simulink model "AltitudeControl"  (Simulink 7.2)
settings: Solver=ode45  StartTime=0.0  StopTime=10.0  RelTol=1e-3
undefined symbols (not defined in the file): DiscIntNeverNeededParam
settings Model: Creator=teme  LastModifiedBy=arnaud
settings OptimizationCC: ExpressionDepthLimit=128
settings DebuggingCC: FcnCallInpInsideContextMsg=Enable All  StrictBusMsg=ErrorLevel1
settings CodeAppCC: CustomSymbolStrType=$N$R$M_T

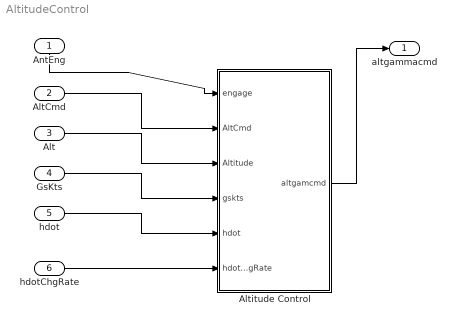
== system AltitudeControl ==
  AntEng : Inport  Orientation=down  DataType=boolean  OutDataTypeStr=boolean
  AltCmd : Inport  Port=2  DataType=double  OutDataTypeStr=double
  Alt : Inport  Port=3  DataType=double  OutDataTypeStr=double
  GsKts : Inport  Port=4  DataType=double  OutDataTypeStr=double
  hdot : Inport  Port=5  DataType=double  OutDataTypeStr=double
  hdotChgRate : Inport  Port=6  DataType=double  OutDataTypeStr=double
  Altitude Control : Subsystem  RequirementInfo={'other' '..\..\tcm_requirements.docx' '@Simulink_requirement_item_14' 'true' 'Altitude Control' '' } %GIDa_5c8df5fb_afa0_485e_88ca_9eaabd9d0f8f
  altgammacmd : Outport
  wires:
  Alt/1 -> Altitude Control/3(Altitude)
  AltCmd/1 -> Altitude Control/2(AltCmd)
  Altitude Control/1(altgamcmd) -> altgammacmd/1
  hdot/1 -> Altitude Control/5(hdot)
  GsKts/1 -> Altitude Control/4(gskts)
  AntEng/1 -> Altitude Control/1(engage)
  hdotChgRate/1 -> Altitude Control/6(hdotChgRate)

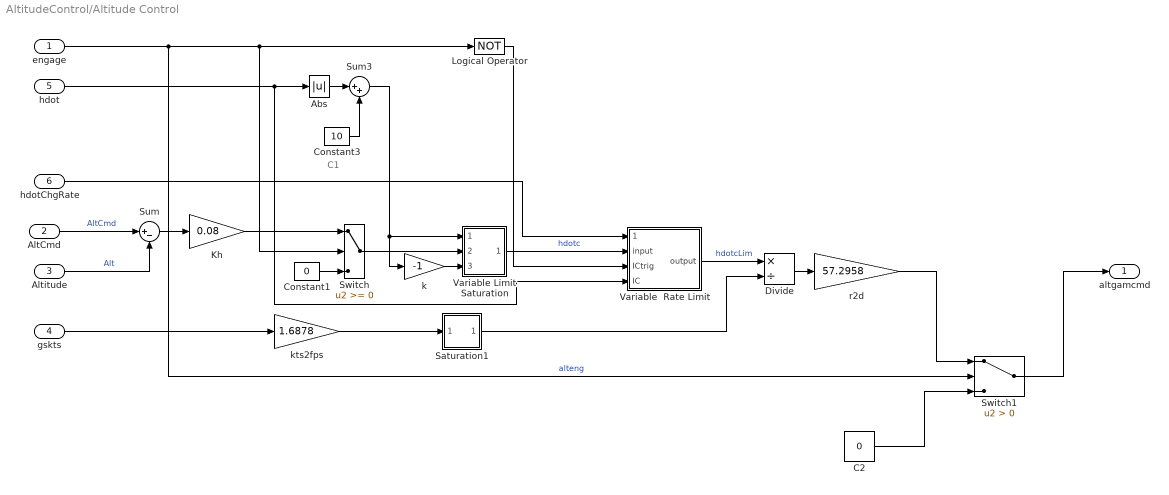
== system AltitudeControl/Altitude Control ==
  note: C1
  engage : Inport  RequirementInfo={} %GIDa_0e288978_810b_404d_8e3d_cfce00b6b13e
  AltCmd : Inport  RequirementInfo={} %GIDa_0cb28106_5eef_4f57_b895_6f6cc316bc91  Port=2
  Altitude : Inport  RequirementInfo={} %GIDa_9d659266_d3a1_41f7_8443_512a58352a3d  Port=3
  gskts : Inport  RequirementInfo={} %GIDa_63cbdc79_cc3a_41e8_a25c_03f8123eb444  Port=4
  hdot : Inport  RequirementInfo={} %GIDa_f80cf171_2707_4e4f_8e83_784456bc38b4  Port=5
  hdotChgRate : Inport  Port=6
  Abs : Abs  RequirementInfo={} %GIDa_20990742_0e4c_4a42_9d74_05382c3e5e10  SaturateOnIntegerOverflow=on
  C2 : Constant  Value=0
  Constant1 : Constant  RequirementInfo={} %GIDa_dca6c410_f388_4f73_ad77_90690c1c79ec  Value=0
  Constant3 : Constant  RequirementInfo={} %GIDa_4d484c55_e80b_4edf_b935_4d0b84fcef43  Value=10
  Divide : Product  RequirementInfo={} %GIDa_a21511b8_8e46_4269_9008_ba9a73618299  Inputs=*/
  Kh : Gain  RequirementInfo={} %GIDa_78bba325_b998_4ee3_b904_8fb0a7f7f7a7  Gain=0.08
  Logical Operator : Logic  RequirementInfo={} %GIDa_3db4e860_846f_470a_babf_a996fcc4fa8f  Operator=NOT
  Saturation1 : Subsystem  RequirementInfo={} %GIDa_f2f227d4_0c3d_4202_a816_beb06b8fee84  TreatAsAtomicUnit=on
  Sum : Sum  RequirementInfo={} %GIDa_c2c23c63_6291_4bac_a67f_cece50fd07b3  Inputs=|+-
  Sum3 : Sum  RequirementInfo={} %GIDa_abda5f80_1075_4cc6_bfe7_9e1cade77fe9  Inputs=|++  SaturateOnIntegerOverflow=on  InputSameDT=on  OutDataTypeStr=Inherit: Same as first input
  Switch : Switch  RequirementInfo={} %GIDa_a81bded5_11a5_4d9b_8d99_08187593493d
  Switch1 : Switch  Criteria=u2 > Threshold
  Variable  Rate Limit : Subsystem  RequirementInfo={} %GIDa_ca745fb3_1ac0_4f87_9ddc_ec0222d57c6c  TreatAsAtomicUnit=on
  Variable Limit Saturation : Subsystem  RequirementInfo={} %GIDa_ceaf2ff3_d3d5_4139_ac40_0e8f5fb26a06  TreatAsAtomicUnit=on
  k : Gain  RequirementInfo={} %GIDa_44367ca2_97f6_4cb9_9c49_9c779fdc721d  Gain=-1
  kts2fps : Gain  RequirementInfo={} %GIDa_8207b08e_fddf_4c38_87c9_e2cb216813f3  Gain=1.6878
  r2d : Gain  RequirementInfo={} %GIDa_573f61a6_cdca_472b_9b49_60142d70b114  Gain=57.2958
  altgamcmd : Outport  RequirementInfo={} %GIDa_cfdf8567_1bf1_487f_8025_1fae61c9e97a
  wires:
  Sum/1 -> Kh/1
  AltCmd/1 -> Sum/1  "AltCmd"
  Altitude/1 -> Sum/2  "Alt"
  hdot/1 -> Variable  Rate Limit/4(IC), Abs/1
  Abs/1 -> Sum3/1
  Constant3/1 -> Sum3/2
  k/1 -> Variable Limit Saturation/3(Lo_lim)
  Sum3/1 -> k/1, Variable Limit Saturation/1(up_lim)
  engage/1 -> Switch1/2, Switch/2, Logical Operator/1  "alteng"
  gskts/1 -> kts2fps/1
  Divide/1 -> r2d/1
  r2d/1 -> Switch1/1
  Logical Operator/1 -> Variable  Rate Limit/3(ICtrig)
  Variable Limit Saturation/1(Out1) -> Variable  Rate Limit/2(input)  "hdotc"
  hdotChgRate/1 -> Variable  Rate Limit/1(ratelim)
  Variable  Rate Limit/1(output) -> Divide/1  "hdotcLim"
  kts2fps/1 -> Saturation1/1(SigIn)
  Saturation1/1(Out1) -> Divide/2
  Switch/1 -> Variable Limit Saturation/2(SigIn)
  Kh/1 -> Switch/1
  Constant1/1 -> Switch/3
  Switch1/1 -> altgamcmd/1
  C2/1 -> Switch1/3

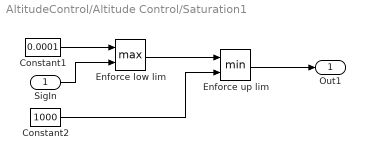
== system AltitudeControl/Altitude Control/Saturation1 ==
  SigIn : Inport  RequirementInfo={} %GIDa_3f5a5311_8185_423f_bf45_67fce5708cdf
  Constant1 : Constant  RequirementInfo={} %GIDa_5a314e61_37a6_49c9_8286_17afee39489d  Value=0.0001
  Constant2 : Constant  RequirementInfo={} %GIDa_19bb776a_128d_4f79_8f32_c6db1286f54e  Value=1000
  Enforce low lim : MinMax  RequirementInfo={} %GIDa_f1ed7bfa_f6af_4dde_ac1b_3ccc756e151e  Function=max  Inputs=2
  Enforce up lim : MinMax  RequirementInfo={} %GIDa_b7d41d07_03e7_4646_9c0d_3c39819752e0  Inputs=2
  Out1 : Outport  RequirementInfo={} %GIDa_a8215b4d_1c2e_47f3_a8fe_a5ea2625158e
  wires:
  Constant1/1 -> Enforce low lim/1
  SigIn/1 -> Enforce low lim/2
  Enforce low lim/1 -> Enforce up lim/1
  Constant2/1 -> Enforce up lim/2
  Enforce up lim/1 -> Out1/1

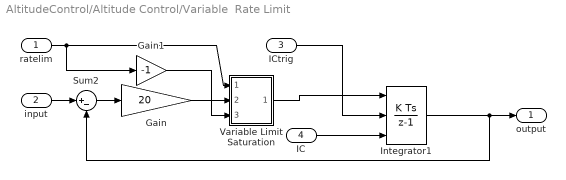
== system AltitudeControl/Altitude Control/Variable  Rate Limit ==
  ratelim : Inport  RequirementInfo={} %GIDa_8a409414_085c_4019_8b8a_edbb028e09c9
  input : Inport  RequirementInfo={} %GIDa_36ca4060_62d0_4794_bfac_efaeb948570f  Port=2  DataType=double  OutDataTypeStr=double
  ICtrig : Inport  RequirementInfo={} %GIDa_210448ec_8901_4d8b_9ae7_bf6603d5175a  Port=3
  IC : Inport  RequirementInfo={} %GIDa_ed78ca41_0e9a_442c_9ce9_efe3f633ea2f  Port=4
  Gain : Gain  RequirementInfo={} %GIDa_8ea2875b_9460_4c83_af15_3f6a067463fd  Gain=20  SaturateOnIntegerOverflow=on  OutDataTypeStr=Inherit: Same as input  ParamDataTypeStr=Inherit: Same as input
  Gain1 : Gain  RequirementInfo={} %GIDa_d92d949d_b0f7_438c_933d_85950dded665  Gain=-1  SaturateOnIntegerOverflow=on  OutDataTypeStr=Inherit: Same as input  ParamDataTypeStr=Inherit: Same as input
  Integrator1 : DiscreteIntegrator  ExternalReset=level  InitialConditionSource=external  SampleTime=0.1  ICPrevOutput=DiscIntNeverNeededParam  ICPrevScaledInput=DiscIntNeverNeededParam  mask(DiscretizedDiscreteIntegrator){}
      mask init:
      | %zoh
  Sum2 : Sum  RequirementInfo={} %GIDa_b334e623_37fe_4ac9_8a97_87088e45dc39  Inputs=|+-  SaturateOnIntegerOverflow=on
  Variable Limit Saturation : Subsystem  RequirementInfo={} %GIDa_455ee4b2_c105_48a1_b2ff_6f4ef26a2acf  TreatAsAtomicUnit=on
  output : Outport  RequirementInfo={} %GIDa_986bb623_f504_4c3d_99b4_2d7370fadfb9
  wires:
  Sum2/1 -> Gain/1
  Gain/1 -> Variable Limit Saturation/2(SigIn)
  ratelim/1 -> Gain1/1, Variable Limit Saturation/1(up_lim)
  Gain1/1 -> Variable Limit Saturation/3(Lo_lim)
  Integrator1/1 -> Sum2/2, output/1
  input/1 -> Sum2/1
  ICtrig/1 -> Integrator1/2
  IC/1 -> Integrator1/3
  Variable Limit Saturation/1(Out1) -> Integrator1/1

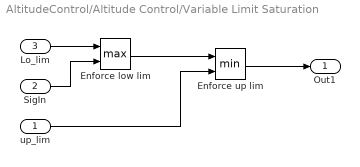
== system AltitudeControl/Altitude Control/Variable Limit Saturation ==
  up_lim : Inport  RequirementInfo={} %GIDa_2e88107a_170e_4209_87ba_bbf099e30048
  SigIn : Inport  RequirementInfo={} %GIDa_1009f7fd_18d1_47a6_bfe8_961b0527e63f  Port=2
  Lo_lim : Inport  RequirementInfo={} %GIDa_25d3a119_7934_4f14_885f_e425c054d3b7  Port=3
  Enforce low lim : MinMax  RequirementInfo={} %GIDa_569de777_726d_4b4c_9368_c3dc4036e8ed  Function=max  Inputs=2
  Enforce up lim : MinMax  RequirementInfo={} %GIDa_08ef4c7c_041a_47cf_8bce_d060e85fd321  Inputs=2
  Out1 : Outport  RequirementInfo={} %GIDa_e97969f5_319c_4569_953d_3be8dc8cd68b
  wires:
  Lo_lim/1 -> Enforce low lim/1
  SigIn/1 -> Enforce low lim/2
  Enforce low lim/1 -> Enforce up lim/1
  up_lim/1 -> Enforce up lim/2
  Enforce up lim/1 -> Out1/1

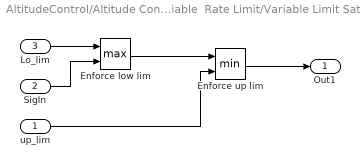
== system AltitudeControl/Altitude Control/Variable  Rate Limit/Variable Limit Saturation ==
  up_lim : Inport  RequirementInfo={} %GIDa_253765a1_7361_4d78_8d4d_1b11f15ce2fa
  SigIn : Inport  RequirementInfo={} %GIDa_df6737d0_f7fe_4781_af6c_3ea749d3e5de  Port=2
  Lo_lim : Inport  RequirementInfo={} %GIDa_c8822ea1_e967_4622_a20b_57b5cefb7799  Port=3
  Enforce low lim : MinMax  RequirementInfo={} %GIDa_fd2a26e9_6c43_40d9_92a2_3b773c237580  Function=max  Inputs=2
  Enforce up lim : MinMax  RequirementInfo={} %GIDa_ef782b40_f42e_44f8_8e6f_8bce9bd7a3f3  Inputs=2
  Out1 : Outport  RequirementInfo={} %GIDa_dbecd57e_14da_4974_8aa6_dc0e6b8a6b18
  wires:
  Enforce up lim/1 -> Out1/1
  up_lim/1 -> Enforce up lim/2
  Enforce low lim/1 -> Enforce up lim/1
  SigIn/1 -> Enforce low lim/2
  Lo_lim/1 -> Enforce low lim/1
